simulink model "HVDC_MMC1_EMT"  (R2023b)
settings: Solver=ode23tb  StartTime=0.0  StopTime=10  MaxStep=Ts  RelTol=1e-3  EnableMultiTasking=on
PreLoadFcn:
  | HVDC_MMC_param
StartFcn:
  | tic
StopFcn:
  | toc
values from neighbouring files (symbols this model uses):
  acdcV = 1/(Vnom_dc/2*sqrt(3)/sqrt(2)/Vnom_sec)    [HVDC_MMC_param.m]
  C_PM = 1.758e-3    (= 0.001758)    [HVDC_MMC_param.m]
  Carm = 1.0*C_pm/n    (= 0.0002096)    [B2B_HVDC_MMC_Calc.m]    (also in HVDC_MMC_param.m = 4.88333333333e-05)
  DC_cable_C_shunt = 0.1e-6    (= 1e-07)    [HVDC_MMC_param.m]
  DC_cable_R_shunt = 1000    [HVDC_MMC_param.m]
  DCM = 1    [HVDC_MMC_param.m]
  Fn_filter = 1000    [B2B_HVDC_MMC_Calc.m]    (also in HVDC_MMC_param.m)
  Fnom = 50    [HVDC_MMC_param.m]
  HRM = 2    [HVDC_MMC_param.m]
  HrmOrd = N    (= 2)    [B2B_HVDC_MMC_Calc.m]    (also in HVDC_MMC_param.m)
  Ib_ac = (2/3)*Pnom/Vb_ac    [HVDC_MMC_param.m]
  Ib_dc = Pnom/Vb_dc    (= 1501.5015015)    [HVDC_MMC_param.m]
  Ki_CCSC = 50    [HVDC_MMC_param.m]
  Ki_Ireg = 6    [HVDC_MMC_param.m]
  Ki_Preg = 1.0    (= 1)    [HVDC_MMC_param.m]
  Ki_Qreg = 1.0    (= 1)    [HVDC_MMC_param.m]
  Ki_VDCreg = 100    [HVDC_MMC_param.m]
  Kp_CCSC = 0.8    [HVDC_MMC_param.m]
  Kp_Ireg = 0.6    [HVDC_MMC_param.m]
  Kp_Preg = 0.5/3    (= 0.166666666667)    [HVDC_MMC_param.m]
  Kp_Qreg = 0.5/3    (= 0.166666666667)    [HVDC_MMC_param.m]
  Kp_VDCreg = 4    [HVDC_MMC_param.m]
  L_cable = 15e-3    (= 0.015)    [HVDC_MMC_param.m]
  Larm = Larm_pu*(Zb_ac/w)    [HVDC_MMC_param.m]
  Lff = Larm_pu/2+Lxfo    (= 0.195)    [HVDC_MMC_param.m]
  Limits_Ireg = [ 2.0  -2.0]    [HVDC_MMC_param.m]
  Limits_Preg = [ 1.2, 0.8 ]    [HVDC_MMC_param.m]
  Limits_Qreg = [ 0.25, -0.25 ]    [HVDC_MMC_param.m]
  Limits_VDCreg = [ 2.0  -2.0]    [HVDC_MMC_param.m]
  Lxfo = 0.12    [HVDC_MMC_param.m]
  Pac = 0.9    [HVDC_MMC_param.m]
  Pnom = 1000e6    (= 1000000000)    [HVDC_MMC_param.m]
  Qac = 0.2    [HVDC_MMC_param.m]
  QCM = 0    [HVDC_MMC_param.m]
  R_cable = 0.5    [HVDC_MMC_param.m]
  Rarm = Rarm_pu*Zb_ac    [HVDC_MMC_param.m]
  Rff = Rarm_pu/2+Rxfo    (= 0.00375)    [HVDC_MMC_param.m]
  Rxfo = 0.003    [HVDC_MMC_param.m]
  Slope_Pref = 0.5    [HVDC_MMC_param.m]
  Slope_Qref = 0.5    [HVDC_MMC_param.m]
  Slope_Vdc_ref = Vnom_dc/5    (= 133200)    [HVDC_MMC_param.m]
  Tbrk1_On = 0.1    [HVDC_MMC_param.m]
  Tbrk2_On = 1.0    (= 1)    [HVDC_MMC_param.m]
  Tdeblock = 1.5    [HVDC_MMC_param.m]
  Tfault = 9999    [HVDC_MMC_param.m]
  Ton_Converter2 = 3    [HVDC_MMC_param.m]
  Ton_PQreg = 2    [HVDC_MMC_param.m]
  Ton_VDCreg = 1.5    [HVDC_MMC_param.m]
  Ts = Ts_Power    (= 5e-05)    [B2B_HVDC_MMC_Calc.m]    (also in HVDC_MMC_param.m)
  Ts_Control = Ts_Power    (= 5e-05)    [B2B_HVDC_MMC_Calc.m]    (also in HVDC_MMC_param.m)
  Ts_DQN = MultTs*Ts_Power    (= 5e-05)    [B2B_HVDC_MMC_Calc.m]    (also in HVDC_MMC_param.m)
  Ts_EMT = Ts    (= 5e-05)    [HVDC_MMC_param.m]
  Ts_Power = 1*50e-6    (= 5e-05)    [B2B_HVDC_MMC_Calc.m]    (also in HVDC_MMC_param.m)
  Vb_ac = sqrt(2/3)*Vnom_sec    [HVDC_MMC_param.m]
  Vb_dc = Vnom_dc    (= 666000)    [HVDC_MMC_param.m]
  Vc0_PM = 0    [HVDC_MMC_param.m]
  Vnom_dc = 2*Vnom_sec    (= 666000)    [HVDC_MMC_param.m]
  Vnom_prim = 333e3    (= 333000)    [HVDC_MMC_param.m]
  Vnom_sec = 333e3    (= 333000)    [HVDC_MMC_param.m]
  w = 2*pi*f    (= 314.159265359)    [B2B_HVDC_MMC_Calc.m]    (also in HVDC_MMC_param.m)
  Ws = 2*pi*Fnom    (= 314.159265359)    [HVDC_MMC_param.m]
  Zb_ac = Vb_ac/Ib_ac    [HVDC_MMC_param.m]
  Zeta_filter = 1    [B2B_HVDC_MMC_Calc.m]    (also in HVDC_MMC_param.m)
undefined symbols (not defined in the file or in its folder): DCss, DiscIntNeverNeededParam, gcbh, MT, sps_rtmsupport
libraries: DQN_Lib x37, simulink x35, spsCurrentMeasurementLib x24, powerlib_extras x21, slpidlib x14, spsSecondOrderFilterLib x14, spsVoltageMeasurementLib x10, spsSeriesRLCBranchLib x10, spsControlledVoltageSourceLib x9, spsHalfBridgeMMCmodel x7, spsGroundLib x4, spsParallelRLCBranchLib x4
(part 1 of 9)
settings Model: Creator=Pierre  LastModifiedBy=rober
settings SolverCC: ConcurrentTasks=on  AlgebraicLoopSolver=TrustRegion  AutoInsertRateTranBlk=on  InsertRTBMode=Never (minimum delay)
settings DataIOCC: SaveFormat=StructureWithTime  SignalLoggingSaveFormat=ModelDataLogs  SaveOutput=off  SignalLogging=off  DSMLogging=off  SaveTime=off  ReturnWorkspaceOutputs=off
settings OptimizationCC: DefaultParameterBehavior=Inlined  EnhancedBackFolding=on  PassReuseOutputArgsAs=Individual arguments  ExpressionDepthLimit=2147483647  OptimizeBlockOrder=speed  DifferentSizesBufferReuse=on  OptimizationCustomize=off  EfficientTunableParamExpr=on
settings DebuggingCC: UnderspecifiedInitializationDetection=Classic  MergeDetectMultiDrivingBlocksExec=none  SolverPrmCheckMsg=warning  ParameterTunabilityLossMsg=error  FcnCallInpInsideContextMsg=warning  UnconnectedInputMsg=warning  UnconnectedOutputMsg=warning  UnconnectedLineMsg=warning  AllowSymbolicDim=off  StateNameClashWarn=warning  SFUnexpectedBacktrackingDiag=warning  SFNoUnconditionalDefaultTransitionDiag=warning  SFExecutionAtInitializationDiag=none  ArithmeticOperatorsInVariantConditions=warning
settings ModelReferenceCC: EnableRefExpFcnMdlSchedulingChecks=on  PropagateSignalLabelsOutOfModel=off
settings SFSimCC: SimUseLocalCustomCode=off  MATLABDynamicMemAlloc=off  CustomCodeUndefinedFunction=UseInterfaceOnly
settings RTWCC: Description=Create Visual C/C++ Solution File for Embedded Coder  SystemTargetFile=ert.tlc  TemplateMakefile=RTW.MSVCBuild  GenerateReport=on  RTWUseLocalCustomCode=off  IncludeHyperlinkInReport=on  LaunchReport=on  GenerateTraceInfo=on  GenerateTraceReport=on  GenerateTraceReportSl=on  GenerateTraceReportSf=on  GenerateTraceReportEml=on  DLArmComputeVersion=19.05
settings CodeAppCC: ForceParamTrailComments=on  IgnoreCustomStorageClasses=off  OperatorAnnotations=on  SimulinkDataObjDesc=on  SFDataObjDesc=on  InsertBlockDesc=on
settings ERTTargetCC: GenerateSampleERTMain=on  InlinedParameterPlacement=NonHierarchical  ERTCustomFileTemplate=example_file_process.tlc
settings ConfigComp: CovMetricSettings=dw  CovSaveCumulativeToWorkspaceVar=on  CovSaveSingleToWorkspaceVar=on  CovExternalEMLEnable=off
settings SimscapeCC: SimscapeNormalizeSystem=off

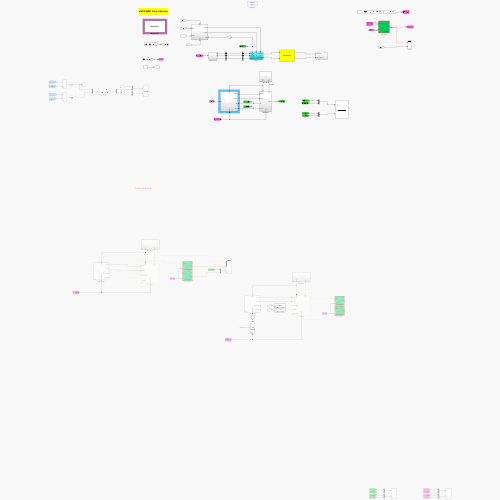
[thumbnail: Simulink's stored preview of the top-level diagram]
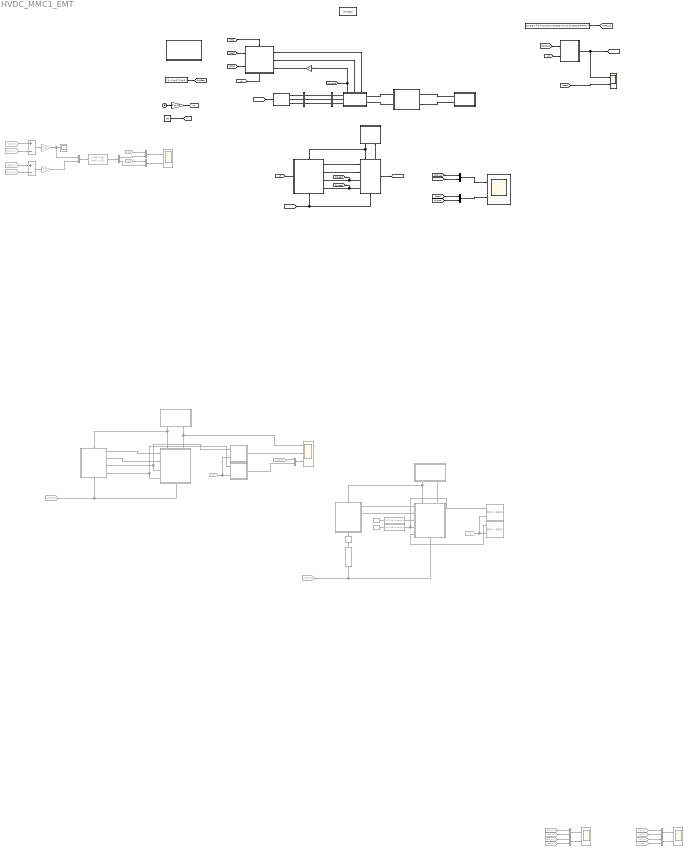
== system HVDC_MMC1_EMT ==
  note: HVDC-MMC Control System
  Add : Sum  Commented=on  Inputs=+-
  Add1 : Sum  Commented=on  Inputs=+-
  CTRL_DQN1 : Subsystem  Commented=on  mask{HarmOrd=HRM}
      mask prompts: HarmOrd "Harmonic order:"
      settings: PortSchema="{\"entries\":[{\"content\":{\"sides\":[{\"content\":{\"connectorIds\":[]},\"type\":\"ConnectorPlacement.EquallySpacedRectSide\",\"uuid\":\"0d082dcb-1cb9-4a87-98e5-35cd432a3a21\"},{\"content\":{\"connectorIds\":[\"Out1\",\"Out2\",\"In3\",\"In4\"],\"side\":\"RIGHT\"},\"type\":\"ConnectorPlacement.EquallySpacedRectSide\",\"uuid\":\"d6c14327-33b3-4ee6-a1e0-7651c9b95832\"},{\"content\":{\"connectorIds\":[\"In1\"],\"side\":\"TOP\"},\"type\":\"ConnectorPlacement.EquallySpacedRectSide\",\"uuid\":\"6be6102f-c019-430a-8225-c31cf73f3a4d\"},{\"content\":{\"connectorIds\":[\"In2\"],\"side\":\"BOTTOM\"},\"type\":\"ConnectorPlacement.EquallySpacedRectSide\",\"uuid\":\"0001f10d-d46a-487c-af5a-06cf58c2ee1d\"}]},\"type\":\"ConnectorPlacement.EquallySpacedConnector\",\"uuid\":\"6102694e-9904-4f4a-845e-781e1c53da4b\"}],\"packageUris\":[\"http://schema.mathworks.com/mf0/Connector/R2020b\"],\"version\":\"1.0\"}"
  CTRL_DQN3 : Subsystem  Commented=on  mask{HarmOrd=HRM}
      mask prompts: HarmOrd "Harmonic order:"
      settings: PortSchema="{\"entries\":[{\"content\":{\"sides\":[{\"content\":{\"connectorIds\":[]},\"type\":\"ConnectorPlacement.EquallySpacedRectSide\",\"uuid\":\"0d082dcb-1cb9-4a87-98e5-35cd432a3a21\"},{\"content\":{\"connectorIds\":[\"Out1\",\"Out2\",\"In3\",\"In4\"],\"side\":\"RIGHT\"},\"type\":\"ConnectorPlacement.EquallySpacedRectSide\",\"uuid\":\"d6c14327-33b3-4ee6-a1e0-7651c9b95832\"},{\"content\":{\"connectorIds\":[\"In1\"],\"side\":\"TOP\"},\"type\":\"ConnectorPlacement.EquallySpacedRectSide\",\"uuid\":\"6be6102f-c019-430a-8225-c31cf73f3a4d\"},{\"content\":{\"connectorIds\":[\"In2\"],\"side\":\"BOTTOM\"},\"type\":\"ConnectorPlacement.EquallySpacedRectSide\",\"uuid\":\"0001f10d-d46a-487c-af5a-06cf58c2ee1d\"}]},\"type\":\"ConnectorPlacement.EquallySpacedConnector\",\"uuid\":\"6102694e-9904-4f4a-845e-781e1c53da4b\"}],\"packageUris\":[\"http://schema.mathworks.com/mf0/Connector/R2020b\"],\"version\":\"1.0\"}"
  Clock : Clock
  Constant1 : Constant  Value="[ 0  -2*pi/3  2*pi/3 ]"  SampleTime=-1
  Constant3 : Constant  Value=complex( [[ 0 Vnom_prim*sqrt(2/3); 0 0; 0 0] zeros(3,HRM-1) ])
  DC Circuit1 : Subsystem
      mask Display: disp('DC circuit')
  DC circuit : StateSpace  Commented=on  A=DCss.A  B=DCss.B  C=DCss.C  D=DCss.D  InitialCondition=DCss.x0
  DC_ABC : Subsystem
      settings: PortSchema="{\"entries\":[{\"content\":{\"sides\":[{\"content\":{\"connectorIds\":[]},\"type\":\"ConnectorPlacement.EquallySpacedRectSide\",\"uuid\":\"5f9f81b4-6131-4450-96fc-72212a851b46\"},{\"content\":{\"connectorIds\":[],\"side\":\"RIGHT\"},\"type\":\"ConnectorPlacement.EquallySpacedRectSide\",\"uuid\":\"0f788077-5580-4ce6-8a1f-7a09e9370e5a\"},{\"content\":{\"connectorIds\":[],\"side\":\"TOP\"},\"type\":\"ConnectorPlacement.EquallySpacedRectSide\",\"uuid\":\"37f0a42c-2dd3-49bf-9631-153ec1fd1df0\"},{\"content\":{\"connectorIds\":[\"In1\",\"Out1\"],\"side\":\"BOTTOM\"},\"type\":\"ConnectorPlacement.EquallySpacedRectSide\",\"uuid\":\"4a78dd89-41c9-4db8-9bc2-9f49ec3f0c10\"}]},\"type\":\"ConnectorPlacement.EquallySpacedConnector\",\"uuid\":\"5112b42b-f0ed-441a-b745-2a1f4f5dce4a\"}],\"packageUris\":[\"http://schema.mathworks.com/mf0/Connector/19700101\"],\"version\":\"1.0\"}"
  DC_ABC1 : Subsystem  Commented=on
      settings: PortSchema="{\"entries\":[{\"content\":{\"sides\":[{\"content\":{\"connectorIds\":[]},\"type\":\"ConnectorPlacement.EquallySpacedRectSide\",\"uuid\":\"5f9f81b4-6131-4450-96fc-72212a851b46\"},{\"content\":{\"connectorIds\":[],\"side\":\"RIGHT\"},\"type\":\"ConnectorPlacement.EquallySpacedRectSide\",\"uuid\":\"0f788077-5580-4ce6-8a1f-7a09e9370e5a\"},{\"content\":{\"connectorIds\":[],\"side\":\"TOP\"},\"type\":\"ConnectorPlacement.EquallySpacedRectSide\",\"uuid\":\"37f0a42c-2dd3-49bf-9631-153ec1fd1df0\"},{\"content\":{\"connectorIds\":[\"In1\",\"Out1\"],\"side\":\"BOTTOM\"},\"type\":\"ConnectorPlacement.EquallySpacedRectSide\",\"uuid\":\"4a78dd89-41c9-4db8-9bc2-9f49ec3f0c10\"}]},\"type\":\"ConnectorPlacement.EquallySpacedConnector\",\"uuid\":\"5112b42b-f0ed-441a-b745-2a1f4f5dce4a\"}],\"packageUris\":[\"http://schema.mathworks.com/mf0/Connector/R2020b\"],\"version\":\"1.0\"}"
  DC_ABC2 : Subsystem  Commented=on
      settings: PortSchema="{\"entries\":[{\"content\":{\"sides\":[{\"content\":{\"connectorIds\":[]},\"type\":\"ConnectorPlacement.EquallySpacedRectSide\",\"uuid\":\"5f9f81b4-6131-4450-96fc-72212a851b46\"},{\"content\":{\"connectorIds\":[],\"side\":\"RIGHT\"},\"type\":\"ConnectorPlacement.EquallySpacedRectSide\",\"uuid\":\"0f788077-5580-4ce6-8a1f-7a09e9370e5a\"},{\"content\":{\"connectorIds\":[],\"side\":\"TOP\"},\"type\":\"ConnectorPlacement.EquallySpacedRectSide\",\"uuid\":\"37f0a42c-2dd3-49bf-9631-153ec1fd1df0\"},{\"content\":{\"connectorIds\":[\"In1\",\"Out1\"],\"side\":\"BOTTOM\"},\"type\":\"ConnectorPlacement.EquallySpacedRectSide\",\"uuid\":\"4a78dd89-41c9-4db8-9bc2-9f49ec3f0c10\"}]},\"type\":\"ConnectorPlacement.EquallySpacedConnector\",\"uuid\":\"5112b42b-f0ed-441a-b745-2a1f4f5dce4a\"}],\"packageUris\":[\"http://schema.mathworks.com/mf0/Connector/R2020b\"],\"version\":\"1.0\"}"
  DQn->ABC : MATLAB Function  TreatAsAtomicUnit=on  SystemSampleTime=Ts  mask{N=HRM}
      mask prompts: N "Harmonic order:"
  DQn->ABC1 : DQN_Lib/DQn->ABC6  Commented=on  N=HrmOrd
  DQn->ABC2 : MATLAB Function  Commented=on  TreatAsAtomicUnit=on  SystemSampleTime=Ts  mask{N=HrmOrd}
      mask prompts: N "Harmonic order:"
  DQn->ABC3 : MATLAB Function  Commented=on  TreatAsAtomicUnit=on  SystemSampleTime=Ts  mask{N=HrmOrd}
      mask prompts: N "Harmonic order:"
  DQn->ABC9 : DQN_Lib/DQn->ABC6  Commented=on  N=HrmOrd
  Demux : Demux  Commented=on  Outputs=2
  From : From  Commented=on  GotoTag=Vdc1  TagVisibility=global
  From1 : From  Commented=on  GotoTag=wt  TagVisibility=global
  From17 : From  Commented=on  GotoTag=Idc_plus  TagVisibility=global
  From19 : From  Commented=on  GotoTag=Idc_minus  TagVisibility=global
  From20 : From  Commented=on  GotoTag=Irec_minus  TagVisibility=global
  From23 : From  Commented=on  GotoTag=Irec_plus  TagVisibility=global
  From24 : From  Commented=on  GotoTag=Vdc2  TagVisibility=global
  From27 : From  Commented=on  GotoTag=Idiff_d2_c  TagVisibility=global
  From30 : From  Commented=on  GotoTag=wt  TagVisibility=global
  From52 : From  Commented=on  GotoTag=Idiff_q2_c  TagVisibility=global
  From53 : From  Commented=on  GotoTag=Idiff_q2  TagVisibility=global
  From55 : From  Commented=on  GotoTag=Idiff_d2  TagVisibility=global
  From56 : From  Commented=on  GotoTag=Md2_c  TagVisibility=global
  From57 : From  Commented=on  GotoTag=Mq2_c  TagVisibility=global
  From58 : From  Commented=on  GotoTag=Md2  TagVisibility=global
  From59 : From  Commented=on  GotoTag=Mq2  TagVisibility=global
  From6 : From  Commented=on  GotoTag=VSRC_C
  From7 : From  Commented=on  GotoTag=Id_abc
  From9 : From  Commented=on  GotoTag=VSRC_C
  Gain : Gain  Gain=2*pi*50
  Gain1 : Gain  Gain=-1
  Gain2 : Gain  Commented=on  Gain=-0.5
  Gain3 : Gain  Commented=on  Gain=0.5
  MATLAB Function1 : DQN_Lib/MATLAB Function4  Commented=on  SystemSampleTime=-1  VariantActivationTime=update diagram  AllowFlexibleInterface=on  Latency=0  AutoFrameSizeCalculation=off
  MATLAB Function2 : DQN_Lib/MATLAB Function4  Commented=on  SystemSampleTime=-1  VariantActivationTime=update diagram  AllowFlexibleInterface=on  Latency=0  AutoFrameSizeCalculation=off
  MATLAB Function9 : DQN_Lib/MATLAB Function4  Commented=on  SystemSampleTime=-1  VariantActivationTime=update diagram  AllowFlexibleInterface=on  Latency=0  AutoFrameSizeCalculation=off
  MMC : Subsystem
      settings: PortSchema="{\"entries\":[{\"content\":{\"sides\":[{\"content\":{\"connectorIds\":[\"LConn1\",\"LConn2\",\"LConn3\"]},\"type\":\"ConnectorPlacement.EquallySpacedRectSide\",\"uuid\":\"74479f40-f186-427a-9533-cd542da214a9\"},{\"content\":{\"connectorIds\":[\"RConn1\",\"RConn2\"],\"side\":\"RIGHT\"},\"type\":\"ConnectorPlacement.EquallySpacedRectSide\",\"uuid\":\"af2aab5a-8cfc-47b9-a3d5-dec541285526\"},{\"content\":{\"connectorIds\":[\"Out1\",\"In1\",\"In2\"],\"side\":\"TOP\"},\"type\":\"ConnectorPlacement.EquallySpacedRectSide\",\"uuid\":\"775fe849-b2f4-496e-a9c1-c2c8ec805134\"}]},\"type\":\"ConnectorPlacement.EquallySpacedConnector\",\"uuid\":\"59d7b4d4-c63b-4498-b4b5-ac9188fab092\"}],\"packageUris\":[\"http://schema.mathworks.com/mf0/Connector/R2020b\"],\"version\":\"1.0\"}"
  MMC_ABC : Subsystem
      settings: PortSchema="{\"entries\":[{\"content\":{\"sides\":[{\"content\":{\"connectorIds\":[\"In1\",\"In2\",\"Out3\",\"Out4\"]},\"type\":\"ConnectorPlacement.EquallySpacedRectSide\",\"uuid\":\"684906a0-21fb-41a6-b3c5-f77045d253ac\"},{\"content\":{\"connectorIds\":[\"Out1\"],\"side\":\"RIGHT\"},\"type\":\"ConnectorPlacement.EquallySpacedRectSide\",\"uuid\":\"9d85a733-ae48-4655-9ff6-63838a16e886\"},{\"content\":{\"connectorIds\":[\"In3\",\"Out2\"],\"side\":\"TOP\"},\"type\":\"ConnectorPlacement.EquallySpacedRectSide\",\"uuid\":\"d076c62e-607a-4519-bbe3-5591fb02f9d6\"},{\"content\":{\"connectorIds\":[\"In4\"],\"side\":\"BOTTOM\"},\"type\":\"ConnectorPlacement.EquallySpacedRectSide\",\"uuid\":\"e22e3e72-7b47-4480-8e5d-6e636dd9340b\"}]},\"type\":\"ConnectorPlacement.EquallySpacedConnector\",\"uuid\":\"6c134aa3-44e6-4e9e-9485-00d5bee37874\"}],\"packageUris\":[\"http://schema.mathworks.com/mf0/Connector/R2020b\"],\"version\":\"1.0\"}"
  MMC_DQN : Subsystem  Commented=on  mask{HrmOrd=HRM, AngFreq=Ws, TimeStep=Ts_DQN}
      mask prompts: HrmOrd "Harmonic order:"; AngFreq "Angular frequency (rad/s):"; TimeStep "Time step (s):"
      settings: PortSchema="{\"entries\":[{\"content\":{\"sides\":[{\"content\":{\"connectorIds\":[\"In1\",\"In2\",\"Out2\",\"Out3\",\"Out4\"]},\"type\":\"ConnectorPlacement.EquallySpacedRectSide\",\"uuid\":\"f639eebb-f91d-4893-aa5c-614953e50141\"},{\"content\":{\"connectorIds\":[],\"side\":\"RIGHT\"},\"type\":\"ConnectorPlacement.EquallySpacedRectSide\",\"uuid\":\"a5873f74-8648-46cb-b48a-fb2ca776885a\"},{\"content\":{\"connectorIds\":[\"In3\",\"Out1\"],\"side\":\"TOP\"},\"type\":\"ConnectorPlacement.EquallySpacedRectSide\",\"uuid\":\"7f3a2d41-300e-41de-a385-bf2dc4de27d8\"},{\"content\":{\"connectorIds\":[\"In4\"],\"side\":\"BOTTOM\"},\"type\":\"ConnectorPlacement.EquallySpacedRectSide\",\"uuid\":\"dc3c6aa9-7c8d-4c08-aa50-6213fc2a18de\"}]},\"type\":\"ConnectorPlacement.EquallySpacedConnector\",\"uuid\":\"a22dadcf-e226-432e-bcde-0bea34be45da\"}],\"packageUris\":[\"http://schema.mathworks.com/mf0/Connector/R2020b\"],\"version\":\"1.0\"}"
  MMC_DQN1 : Subsystem  Commented=on  mask{HrmOrd=HRM, AngFreq=Ws, TimeStep=Ts_DQN}
      mask prompts: HrmOrd "Harmonic order:"; AngFreq "Angular frequency (rad/s):"; TimeStep "Time step (s):"
      settings: PortSchema="{\"entries\":[{\"content\":{\"sides\":[{\"content\":{\"connectorIds\":[\"In1\",\"In2\",\"Out2\",\"Out3\"]},\"type\":\"ConnectorPlacement.EquallySpacedRectSide\",\"uuid\":\"f639eebb-f91d-4893-aa5c-614953e50141\"},{\"content\":{\"side\":\"RIGHT\"},\"type\":\"ConnectorPlacement.EquallySpacedRectSide\",\"uuid\":\"a5873f74-8648-46cb-b48a-fb2ca776885a\"},{\"content\":{\"connectorIds\":[\"In3\",\"Out1\"],\"side\":\"TOP\"},\"type\":\"ConnectorPlacement.EquallySpacedRectSide\",\"uuid\":\"7f3a2d41-300e-41de-a385-bf2dc4de27d8\"},{\"content\":{\"connectorIds\":[\"In4\"],\"side\":\"BOTTOM\"},\"type\":\"ConnectorPlacement.EquallySpacedRectSide\",\"uuid\":\"dc3c6aa9-7c8d-4c08-aa50-6213fc2a18de\"}]},\"type\":\"ConnectorPlacement.EquallySpacedConnector\",\"uuid\":\"a22dadcf-e226-432e-bcde-0bea34be45da\"}],\"packageUris\":[\"http://schema.mathworks.com/mf0/Connector/R2020b\"],\"version\":\"1.0\"}"
  Mux{,1..3,15..18} (8 alike) : Mux  Commented=on  Inputs=2
  Mux4 : Mux  Inputs=2
  Mux5 : Mux  Inputs=2
  Pi1 : Constant  Value=50  OutDataTypeStr=Inherit: Inherit via back propagation
  Reshape : Reshape  Commented=on
  Reshape1 : Reshape  Commented=on
  Reshape2 : Reshape  Commented=on
  Scope : Scope  NumInputPorts=2
  Scope1 : Scope  NumInputPorts=2
  Scope10 : Scope  Commented=on  NumInputPorts=2
  Scope2 : Scope  Commented=on  NumInputPorts=3
  Scope3 : Scope  Commented=on
  Scope4 : Scope  Commented=on  NumInputPorts=2
  Scope9 : Scope  Commented=on  NumInputPorts=2
  Sequencer : Subsystem
      mask Display: disp('Sequencer')
  Subsystem : Subsystem
      settings: PortSchema="{\"entries\":[{\"content\":{\"sides\":[{\"content\":{\"connectorIds\":[\"In1\"]},\"type\":\"ConnectorPlacement.EquallySpacedRectSide\",\"uuid\":\"0eb80377-11e9-4327-8c94-fb94b1ae678e\"},{\"content\":{\"connectorIds\":[\"Out1\",\"Out2\",\"In4\",\"In5\"],\"side\":\"RIGHT\"},\"type\":\"ConnectorPlacement.EquallySpacedRectSide\",\"uuid\":\"6596dc6b-6b23-47fc-bea2-6996abd2ba15\"},{\"content\":{\"connectorIds\":[\"In2\"],\"side\":\"TOP\"},\"type\":\"ConnectorPlacement.EquallySpacedRectSide\",\"uuid\":\"8e21476a-42ed-42f6-8dc5-d6cd1acd5e6a\"},{\"content\":{\"connectorIds\":[\"In3\"],\"side\":\"BOTTOM\"},\"type\":\"ConnectorPlacement.EquallySpacedRectSide\",\"uuid\":\"64f4f9aa-7403-4df9-a838-1dcd5c8e1624\"}]},\"type\":\"ConnectorPlacement.EquallySpacedConnector\",\"uuid\":\"bea88ec7-c79f-4685-875b-b84ad23b5423\"}],\"packageUris\":[\"http://schema.mathworks.com/mf0/Connector/R2020b\"],\"version\":\"1.0\"}"
  Subsystem1 : Subsystem
  Subsystem2 : Subsystem
      settings: PortSchema="{\"entries\":[{\"content\":{\"sides\":[{\"content\":{\"connectorIds\":[\"In1\",\"In2\"]},\"type\":\"ConnectorPlacement.EquallySpacedRectSide\",\"uuid\":\"0eb80377-11e9-4327-8c94-fb94b1ae678e\"},{\"content\":{\"connectorIds\":[\"Out1\",\"Out2\",\"In5\"],\"side\":\"RIGHT\"},\"type\":\"ConnectorPlacement.EquallySpacedRectSide\",\"uuid\":\"6596dc6b-6b23-47fc-bea2-6996abd2ba15\"},{\"content\":{\"connectorIds\":[\"In3\"],\"side\":\"TOP\"},\"type\":\"ConnectorPlacement.EquallySpacedRectSide\",\"uuid\":\"8e21476a-42ed-42f6-8dc5-d6cd1acd5e6a\"},{\"content\":{\"connectorIds\":[\"In4\"],\"side\":\"BOTTOM\"},\"type\":\"ConnectorPlacement.EquallySpacedRectSide\",\"uuid\":\"64f4f9aa-7403-4df9-a838-1dcd5c8e1624\"}]},\"type\":\"ConnectorPlacement.EquallySpacedConnector\",\"uuid\":\"bea88ec7-c79f-4685-875b-b84ad23b5423\"}],\"packageUris\":[\"http://schema.mathworks.com/mf0/Connector/R2020b\"],\"version\":\"1.0\"}"
  Voltage source : Subsystem
  conv : spsThreePhaseVIMeasurementLib/Three-Phase V-I Measurement  VoltageMeasurement=phase-to-ground  SetLabelV=on  LabelV=Vconv  Vpu=off  VpuLL=off  CurrentMeasurement=no  SetLabelI=on  LabelI=Isec  Ipu=off  Pbase=100e6  Vbase=500e3  OutputType=Complex  PhasorSimulation=off  PSBequivalent=0
  powergui : spspowerguiLib/powergui  Priority=1  SimulationMode=Discrete  SampleTime=Ts  frequency=60  Iterations=50  frequencyindice=0  Pbase=100e6  ErrMax=1e-4  UnitsV=kV  UnitsW=MW  buscounter=0  FunctionMessages=off  echomessages=off  EnableUseOfTLC=off  CurrentSourceSwitches=off  DisableSnubberDevices=off  DisableRonSwitches=off  DisableVfSwitches=off  DisplayEquations=off  AutomaticDiscreteSolvers=off  SolverType=Tustin/Backward Euler (TBE)  Interpol=off  ExternalGateDelay=off  methode=off  Ts=100  x0status=blocks  SPID=off  SwTol=0  HookPort=off  NonlinearTolerance=1e-4  nMaxIteration=100  ContinueOnMaxIteration=off  RestoreLinks=warning  ResistiveCurrentMeasurement=off  Frange=[0:2:500]  Ylog=off  Xlog=on  ShowGrid=off  save=off  variable=ZData  structure=ScopeData1  ZoomFFT=off  StartTime=9  cycles=100  DisplayStyle=1  fundamental=50  FreqAxis=off  MaxFrequency=100  frequencyindicesteady=1  RmsSteady=1  display=off
  sec : spsThreePhaseVIMeasurementLib/Three-Phase V-I Measurement  VoltageMeasurement=phase-to-ground  SetLabelV=on  LabelV=Vsec  Vpu=off  VpuLL=off  CurrentMeasurement=yes  SetLabelI=on  LabelI=Isec  Ipu=off  Pbase=100e6  Vbase=500e3  OutputType=Complex  PhasorSimulation=off  PSBequivalent=0
  tag scope: PosSeq=global, f=global, wt=global
  wires:
  Pi1/1 -> [f]
  Gain/1 -> [wt]
  Clock/1 -> Gain/1
  Constant1/1 -> [PosSeq]
  Mux15/1 -> Scope9/1
  Mux16/1 -> Scope9/2
  From55/1 -> Mux15/2
  From27/1 -> Mux15/1
  From53/1 -> Mux16/2
  From52/1 -> Mux16/1
  Mux18/1 -> Scope10/2
  From56/1 -> Mux17/1
  From59/1 -> Mux18/2
  From58/1 -> Mux17/2
  Mux17/1 -> Scope10/1
  From57/1 -> Mux18/1
  [Vsec] -> Scope/2
  [wt] -> DQn->ABC/2(tho)  "theta"
  Constant3/1 -> [VSRC_C]
  [VSRC_C] -> DQn->ABC/1(Xdcpnz_c)  "[N+1,18 (6+6+6)]"
  DQn->ABC/1(Xabc) -> Scope/1, [Vsec_ABC]  "Mac_EMT"
  MMC_ABC/4(Iconv1) -> [Ic_abc], Subsystem/5(Iconv)
  Subsystem/1("{m_dq1}") -> MMC_ABC/1(m_dq1)
  [Vsec_ABC] -> Subsystem/3(Vsec), MMC_ABC/4(Vsec)
  DC_ABC/1(Vdc1) -> Subsystem/2(Vdc), MMC_ABC/3(Vdc)
  [wt] -> Subsystem/1(wt)
  Subsystem/2("{m_dq2}") -> MMC_ABC/2(m_dq2)
  MMC_ABC/2(Idc) -> DC_ABC/1(Idc1)  "Idc_ABC"
  MMC_ABC/3(Id) -> [Id_abc], Subsystem/4(Idiff)
  CTRL_DQN3/1(m_dq1) -> MMC_DQN/1(m_dq1)
  ? -> ?
  DC_ABC1/1(Vdc1) -> CTRL_DQN3/1(Vdc), MMC_DQN/3(Vdc)
  CTRL_DQN3/2(m_dq2) -> MMC_DQN/2(m_dq2)
  From30/1 -> DQn->ABC1/2, DQn->ABC9/2
  From6/1 -> MATLAB Function2/1, MMC_DQN/4(Vs_DQN)
  MMC_DQN/4(Vconv_DQN) -> DQn->ABC1/1
  MMC_DQN/3(Id_DQN) -> DQn->ABC9/1, MATLAB Function1/1
  MMC_DQN/2(Iconv_DQN) -> MATLAB Function9/1
  MMC_DQN/1(Idc) -> DC_ABC1/1(Idc1)
  Subsystem2/2("{m_dq2}") -> MMC/1(m_dq2)
  [Isec] -> Subsystem2/2(Iconv)
  Subsystem2/1("{m_dq1}") -> MMC/2(m_dq1)
  MMC/1(Id_abc) -> Gain1/1, [Id_emt]
  [Vdc1] -> Subsystem2/3(Vdc)
  [Vsec] -> Subsystem2/1(Vsec)
  Gain1/1 -> Subsystem2/5(Idiff)
  [wt] -> Subsystem2/4(wt)
  [Vsec_ABC] -> Voltage source/1(In1)
  MATLAB Function9/1 -> Reshape/1
  MATLAB Function1/1 -> Reshape1/1
  MATLAB Function2/1 -> Reshape2/1
  Reshape2/1 -> CTRL_DQN3/2(Vs_DQN)
  CTRL_DQN1/1(m_dq1) -> MMC_DQN1/1(m_dq1)
  DC_ABC2/1(Vdc1) -> CTRL_DQN1/1(Vdc), MMC_DQN1/3(Vdc)
  CTRL_DQN1/2(m_dq2) -> MMC_DQN1/2(m_dq2)
  MMC_DQN1/1(Idc) -> DC_ABC2/1(Idc1), Scope2/1
  From9/1 -> MMC_DQN1/4(Vs_DQN), CTRL_DQN1/2(Vs_DQN)
  From1/1 -> DQn->ABC2/2(tho), DQn->ABC3/2(tho)
  MMC_DQN1/2(Iconv_DQN) -> DQn->ABC3/1(Xdcpnz_c), CTRL_DQN1/3(Iconv_DQN)
  MMC_DQN1/3(Id_DQN) -> DQn->ABC2/1(Xdcpnz_c), CTRL_DQN1/4(Id_DQN)
  DQn->ABC2/1(Xabc) -> Mux/2
  DQn->ABC3/1(Xabc) -> Scope2/2
  Mux/1 -> Scope2/3
  From7/1 -> Mux/1
  Mux1/1 -> DC circuit/1
  DC circuit/1 -> Demux/1
  From19/1 -> Add/2
  Add/1 -> Gain2/1
  Gain2/1 -> Mux1/1, Scope3/1
  From17/1 -> Add/1
  From23/1 -> Add1/1
  From20/1 -> Add1/2
  Add1/1 -> Gain3/1
  Gain3/1 -> Mux1/2
  Mux2/1 -> Scope4/1
  Mux3/1 -> Scope4/2
  From/1 -> Mux2/1
  Demux/1 -> Mux2/2
  From24/1 -> Mux3/1
  Demux/2 -> Mux3/2
  MMC_ABC/1(Vconv) -> [Vconv_abc]
  [Vconv_abc] -> Mux4/2
  [Ic_abc] -> Mux5/2
  [Isec] -> Mux5/1
  [Vconv] -> Mux4/1
  Mux4/1 -> Scope1/1
  Mux5/1 -> Scope1/2
  connections:
  sec/LConn1 -- conv/RConn1
  Voltage source/RConn3 -- sec/RConn3
  MMC/LConn3 -- conv/LConn3
  sec/LConn3 -- conv/RConn3
  sec/LConn2 -- conv/RConn2
  MMC/LConn1 -- conv/LConn1
  Voltage source/RConn1 -- sec/RConn1
  Voltage source/RConn2 -- sec/RConn2
  MMC/LConn2 -- conv/LConn2
  DC Circuit1/LConn1 -- MMC/RConn1
  DC Circuit1/LConn2 -- MMC/RConn2
  DC Circuit1/RConn1 -- Subsystem1/LConn1
  DC Circuit1/RConn2 -- Subsystem1/LConn2

== system HVDC_MMC1_EMT/CTRL_DQN1 ==
  Vdc : Inport
  Vs_DQN : Inport  Port=2
  Iconv_DQN : Inport  Port=3
  Id_DQN : Inport  Port=4
  I->pu1 : Gain  Gain=1/Ib_ac  SaturateOnIntegerOverflow=on  OutDataTypeStr=Inherit: Same as input  ParamDataTypeStr=Inherit: Same as input
  I->pu13 : Gain  Gain=1/Vb_ac  SaturateOnIntegerOverflow=on  OutDataTypeStr=Inherit: Same as input  ParamDataTypeStr=Inherit: Same as input
  I->pu2 : Gain  Gain=1/Ib_ac  SaturateOnIntegerOverflow=on  OutDataTypeStr=Inherit: Same as input  ParamDataTypeStr=Inherit: Same as input
  MATLAB Function1 : DQN_Lib/MATLAB Function4  SystemSampleTime=-1  VariantActivationTime=update diagram  AllowFlexibleInterface=on  Latency=0  AutoFrameSizeCalculation=off
  MATLAB Function4 : DQN_Lib/MATLAB Function4  SystemSampleTime=-1  VariantActivationTime=update diagram  AllowFlexibleInterface=on  Latency=0  AutoFrameSizeCalculation=off
  MATLAB Function9 : DQN_Lib/MATLAB Function4  SystemSampleTime=-1  VariantActivationTime=update diagram  AllowFlexibleInterface=on  Latency=0  AutoFrameSizeCalculation=off
  Mux1 : Mux  Inputs=2
  Mux3 : Mux  Inputs=2
  Mux4 : Mux  Inputs=2
  Reshape : Reshape
  Reshape1 : Reshape
  Reshape4 : Reshape
  Selector1 : Selector  InputPortWidth=HrmOrd+1  IndexOptions=Index vector (dialog)  Indices=3  OutputSizes=1
  Selector{6..7,9..10} (4 alike) : Selector  InputPortWidth=HrmOrd+1  IndexOptions=Index vector (dialog)  Indices=2  OutputSizes=1
  Selector2 : Selector  InputPortWidth=HrmOrd+1  IndexOptions=Index vector (dialog)  Indices=3  OutputSizes=1
  Subsystem : DQN_Lib/Subsystem  N=HrmOrd
  Subsystem1 : Subsystem  Commented=on
  Subsystem2 : Subsystem  mask{Ts=Ts_DQN, Fnom=Fnom, acdcV=acdcV, Fn_filter=Fn_filter, Zeta_filter=Zeta_filter, Kp_Preg=Kp_Preg, Ki_Preg=Ki_Preg, Limits_Preg_1=Limits_Preg(1), Limits_Preg_2=Limits_Preg(2), Kp_Qreg=Kp_Qreg, Ki_Qreg=Ki_Qreg, Limits_Qreg_1=Limits_Qreg(1), Limits_Qreg_2=Limits_Qreg(2), Kp_VDCreg=Kp_VDCreg, Ki_VDCreg=Ki_VDCreg, Limits_VDCreg_1=Limits_VDCreg(1), Limits_VDCreg_2=Limits_VDCreg(2), Kp_Ireg=Kp_Ireg, Ki_Ireg=Ki_Ireg, Limits_Ireg=Limits_Ireg, Rff=Rff, Lff=Lff, Kp_CCSC=Kp_CCSC, Ki_CCSC=Ki_CCSC}
      mask prompts: Ts "Sample time:"; Fnom "Fundamental frequency (Hz):"; Fn_filter "Natural frequency fn (Hz):"; Zeta_filter "Damping ratio Zeta"; Kp_Preg "Proportional (P):"; Ki_Preg "Integral (I):"; Limits_Preg_1 "Upper limit:"; Limits_Preg_2 "Lower limit:"; Kp_Qreg "Proportional (P):"; Ki_Qreg "Integral (I):"; Limits_Qreg_1 "Upper limit:"; Limits_Qreg_2 "Lower limit:"; Kp_VDCreg "Proportional (P):"; Ki_VDCreg "Integral (I):"; Limits_VDCreg_1 "Upper limit:"; Limits_VDCreg_2 "Lower limit:"; Kp_Ireg "Proportional (P):"; Ki_Ireg "Integral (I):"; Limits_Ireg "Output limits:"; Kp_CCSC "Proportional (P):"; Ki_CCSC "Integral (I):"
      mask DialogControl Container6 Prompt: General
      mask DialogControl Container14 Prompt: Filter
      mask DialogControl Container14_copy Prompt: Active power regulator
      mask DialogControl Container14_copy_copy Prompt: Reactive power regulator
      mask DialogControl Container14_copy_copy_copy Prompt: DC voltage regulator
      mask DialogControl Container14_copy_copy_copy_copy Prompt: Current regulator
      mask DialogControl Container14_copy_copy_copy_copy_copy Prompt: CCSC
  Subsystem4 : DQN_Lib/Subsystem  N=HrmOrd
  Subsystem5 : DQN_Lib/Subsystem  N=HrmOrd
  V->pu1 : Gain  Gain=1/Vb_ac  SaturateOnIntegerOverflow=on  OutDataTypeStr=Inherit: Same as input  ParamDataTypeStr=Inherit: Same as input
  m_dq1 : Outport
  m_dq2 : Outport  Port=2
  wires:
  Subsystem5/4 -> Selector10/1
  Subsystem4/1 -> Selector6/1
  Subsystem4/4 -> Selector7/1
  Subsystem5/1 -> Selector9/1
  V->pu1/1 -> Subsystem5/1
  Reshape4/1 -> V->pu1/1
  Vdc/1 -> I->pu13/1
  Subsystem2/1(m_dq1) -> m_dq1/1
  I->pu2/1 -> Subsystem4/1
  I->pu13/1 -> Subsystem2/1(Vdc)
  Mux4/1 -> Subsystem2/2(Vs_dq1)
  Mux3/1 -> Subsystem2/3(Iconv_dq1)
  Subsystem/5 -> Selector2/1
  I->pu1/1 -> Subsystem/1
  Selector1/1 -> Mux1/1
  Selector2/1 -> Mux1/2
  Mux1/1 -> Subsystem2/4(Id_dq2)
  Subsystem/2 -> Selector1/1
  [PSCC_On] -> Subsystem2/8(PQreg_On1)
  [PQreg_On] -> Subsystem2/5(PQreg_On)
  [VDCreg_On] -> Subsystem2/6(VDCreg_On)
  Selector9/1 -> Mux4/1
  Selector10/1 -> Mux4/2
  Selector6/1 -> Mux3/1
  Selector7/1 -> Mux3/2
  Subsystem2/2(m_dq2) -> m_dq2/1
  [Vdc_ref] -> Subsystem2/7(Vdc_ref)
  MATLAB Function9/1 -> Reshape/1
  MATLAB Function1/1 -> Reshape1/1
  Iconv_DQN/1 -> MATLAB Function9/1
  Reshape/1 -> I->pu2/1
  Id_DQN/1 -> MATLAB Function1/1
  Reshape1/1 -> I->pu1/1
  MATLAB Function4/1 -> Reshape4/1
  Vs_DQN/1 -> MATLAB Function4/1

== system HVDC_MMC1_EMT/CTRL_DQN3 ==
  note: HRM
  note: HRM
  Vdc : Inport
  Vs_DQN : Inport  Port=2
  Iconv_DQN : Inport  Port=3
  Id_DQN : Inport  Port=4
  Demux1 : Demux  Outputs=[HrmOrd+1, HrmOrd+1, HrmOrd+1, HrmOrd+1, HrmOrd+1, HrmOrd+1]
  Demux2 : Demux  Outputs=[HrmOrd+1, HrmOrd+1, HrmOrd+1, HrmOrd+1, HrmOrd+1, HrmOrd+1]
  Demux4 : Demux  Outputs=[HrmOrd+1, HrmOrd+1, HrmOrd+1, HrmOrd+1, HrmOrd+1, HrmOrd+1]
  I->pu1 : Gain  Gain=1/Ib_ac  SaturateOnIntegerOverflow=on  OutDataTypeStr=Inherit: Same as input  ParamDataTypeStr=Inherit: Same as input
  I->pu13 : Gain  Gain=1/Vb_ac  SaturateOnIntegerOverflow=on  OutDataTypeStr=Inherit: Same as input  ParamDataTypeStr=Inherit: Same as input
  I->pu2 : Gain  Gain=1/Ib_ac  SaturateOnIntegerOverflow=on  OutDataTypeStr=Inherit: Same as input  ParamDataTypeStr=Inherit: Same as input
  Mux1 : Mux  Inputs=2
  Mux3 : Mux  Inputs=2
  Mux4 : Mux  Inputs=2
  Selector1 : Selector  InputPortWidth=HrmOrd+1  IndexOptions=Index vector (dialog)  Indices=3  OutputSizes=1
  Selector{6..7,9..10} (4 alike) : Selector  InputPortWidth=HrmOrd+1  IndexOptions=Index vector (dialog)  Indices=2  OutputSizes=1
  Selector2 : Selector  InputPortWidth=HrmOrd+1  IndexOptions=Index vector (dialog)  Indices=3  OutputSizes=1
  Subsystem1 : Subsystem  Commented=on
  Subsystem2 : Subsystem  mask{Ts=Ts_DQN, Fnom=Fnom, acdcV=acdcV, Fn_filter=Fn_filter, Zeta_filter=Zeta_filter, Kp_Preg=Kp_Preg, Ki_Preg=Ki_Preg, Limits_Preg_1=Limits_Preg(1), Limits_Preg_2=Limits_Preg(2), Kp_Qreg=Kp_Qreg, Ki_Qreg=Ki_Qreg, Limits_Qreg_1=Limits_Qreg(1), Limits_Qreg_2=Limits_Qreg(2), Kp_VDCreg=Kp_VDCreg, Ki_VDCreg=Ki_VDCreg, Limits_VDCreg_1=Limits_VDCreg(1), Limits_VDCreg_2=Limits_VDCreg(2), Kp_Ireg=Kp_Ireg, Ki_Ireg=Ki_Ireg, Limits_Ireg=Limits_Ireg, Rff=Rff, Lff=Lff, Kp_CCSC=Kp_CCSC, Ki_CCSC=Ki_CCSC}
      mask prompts: Ts "Sample time:"; Fnom "Fundamental frequency (Hz):"; Fn_filter "Natural frequency fn (Hz):"; Zeta_filter "Damping ratio Zeta"; Kp_Preg "Proportional (P):"; Ki_Preg "Integral (I):"; Limits_Preg_1 "Upper limit:"; Limits_Preg_2 "Lower limit:"; Kp_Qreg "Proportional (P):"; Ki_Qreg "Integral (I):"; Limits_Qreg_1 "Upper limit:"; Limits_Qreg_2 "Lower limit:"; Kp_VDCreg "Proportional (P):"; Ki_VDCreg "Integral (I):"; Limits_VDCreg_1 "Upper limit:"; Limits_VDCreg_2 "Lower limit:"; Kp_Ireg "Proportional (P):"; Ki_Ireg "Integral (I):"; Limits_Ireg "Output limits:"; Kp_CCSC "Proportional (P):"; Ki_CCSC "Integral (I):"
      mask DialogControl Container6 Prompt: General
      mask DialogControl Container14 Prompt: Filter
      mask DialogControl Container14_copy Prompt: Active power regulator
      mask DialogControl Container14_copy_copy Prompt: Reactive power regulator
      mask DialogControl Container14_copy_copy_copy Prompt: DC voltage regulator
      mask DialogControl Container14_copy_copy_copy_copy Prompt: Current regulator
      mask DialogControl Container14_copy_copy_copy_copy_copy Prompt: CCSC
  V->pu1 : Gain  Gain=1/Vb_ac  SaturateOnIntegerOverflow=on  OutDataTypeStr=Inherit: Same as input  ParamDataTypeStr=Inherit: Same as input
  m_dq1 : Outport
  m_dq2 : Outport  Port=2
  wires:
  Demux1/4 -> Selector10/1
  Demux4/1 -> Selector6/1
  Demux4/4 -> Selector7/1
  Demux1/1 -> Selector9/1
  V->pu1/1 -> Demux1/1
  Vs_DQN/1 -> V->pu1/1
  Id_DQN/1 -> I->pu1/1
  Vdc/1 -> I->pu13/1
  Iconv_DQN/1 -> I->pu2/1
  Subsystem2/1(m_dq1) -> m_dq1/1
  I->pu2/1 -> Demux4/1
  I->pu13/1 -> Subsystem2/1(Vdc)
  Mux4/1 -> Subsystem2/2(Vs_dq1)
  Mux3/1 -> Subsystem2/3(Iconv_dq1)
  Demux2/5 -> Selector2/1
  I->pu1/1 -> Demux2/1
  Selector1/1 -> Mux1/1
  Selector2/1 -> Mux1/2
  Mux1/1 -> Subsystem2/4(Id_dq2)
  Demux2/2 -> Selector1/1
  [PSCC_On] -> Subsystem2/8(PQreg_On1)
  [PQreg_On] -> Subsystem2/5(PQreg_On)
  [VDCreg_On] -> Subsystem2/6(VDCreg_On)
  Selector9/1 -> Mux4/1
  Selector10/1 -> Mux4/2
  Selector6/1 -> Mux3/1
  Selector7/1 -> Mux3/2
  Subsystem2/2(m_dq2) -> m_dq2/1
  [Vdc_ref] -> Subsystem2/7(Vdc_ref)

== system HVDC_MMC1_EMT/DC Circuit1 ==
  note: Cable
      | (simplified model)
  Current Measurement2 : spsCurrentMeasurementLib/Current Measurement  PhasorSimulation=off  OutputType=Complex  PSBequivalent=0
  Ground : spsGroundLib/Ground  LConnTagsString=a
  Ground2 : spsGroundLib/Ground  LConnTagsString=a
  Parallel RLC Branch{,1..3} (4 alike) : spsParallelRLCBranchLib/Parallel RLC Branch  LConnTagsString=a  RConnTagsString=__new0  BranchType=RC  Resistance=DC_cable_R_shunt  Inductance=1e-3  SetiL0=off  InitialCurrent=0  Capacitance=DC_cable_C_shunt  Setx0=off  InitialVoltage=0  Measurements=None
  Voltage Measurement2 : spsVoltageMeasurementLib/Voltage Measurement  PhasorSimulation=off  OutputType=Complex  PSBequivalent=0
  Voltage Measurement3 : spsVoltageMeasurementLib/Voltage Measurement  PhasorSimulation=off  OutputType=Complex  PSBequivalent=0
  Zcable1_1 : spsSeriesRLCBranchLib/Series RLC Branch  LConnTagsString=__new0  RConnTagsString=__new0  BranchType=RL  Resistance=R_cable  Inductance=L_cable  SetiL0=off  InitialCurrent=0  Capacitance=1e-6  Setx0=off  InitialVoltage=0  Measurements=None
  Zcable2_1 : spsSeriesRLCBranchLib/Series RLC Branch  LConnTagsString=__new0  RConnTagsString=__new0  BranchType=RL  Resistance=R_cable  Inductance=L_cable  SetiL0=off  InitialCurrent=0  Capacitance=1e-6  Setx0=off  InitialVoltage=0  Measurements=None
  CBL_plus : PMIOPort  Side=Left
  CBL_minus : PMIOPort  Port=2  Side=Left
  CBR_plus : PMIOPort  Port=3  Side=Right
  CBR_minus : PMIOPort  Port=4  Side=Right
  tag scope: Idc1=global, Vdc1=global, Vdc2=global
  wires:
  Voltage Measurement2/1 -> [Vdc1]
  Current Measurement2/1 -> [Idc1]
  Voltage Measurement3/1 -> [Vdc2]
  connections:
  CBL_minus/RConn1 -- Voltage Measurement2/LConn2 -- Zcable2_1/RConn1 -- Parallel RLC Branch1/RConn1
  Zcable1_1/RConn1 -- Voltage Measurement2/LConn1 -- Current Measurement2/LConn1 -- Parallel RLC Branch/LConn1
  Current Measurement2/RConn1 -- CBL_plus/RConn1
  Voltage Measurement3/LConn2 -- Zcable2_1/LConn1 -- CBR_minus/RConn1 -- Parallel RLC Branch3/RConn1
  Parallel RLC Branch/RConn1 -- Ground/LConn1 -- Parallel RLC Branch1/LConn1
  Parallel RLC Branch2/RConn1 -- Ground2/LConn1 -- Parallel RLC Branch3/LConn1
  Voltage Measurement3/LConn1 -- Zcable1_1/LConn1 -- CBR_plus/RConn1 -- Parallel RLC Branch2/LConn1

== system HVDC_MMC1_EMT/DC_ABC ==
  Idc1 : Inport
  Add1 : Sum  Inputs=-+
  Add5 : Sum
  Constant2 : Constant  Value=DCM
  Constant3 : Constant  Value=DCM
  DC Voltage Regulator (VDCreg)2 : Subsystem
  Delay2 : Delay  DelayLength=1
  Discrete Derivative : simulink/Discrete/Discrete Derivative  Commented=on  gainval=1  ICPrevScaledInput=0.0  OutMin=[]  OutMax=[]  OutDataType=fixdt(1, 16)  OutScaling=2^-10  DoSatur=off
  Gain3 : Gain  Gain=R_cable/2
  Gain6 : Gain  Gain=L_cable/2
  I->pu3 : Gain  Gain=1/Ib_dc  SaturateOnIntegerOverflow=on  OutDataTypeStr=Inherit: Same as input  ParamDataTypeStr=Inherit: Same as input
  I->pu5 : Gain  Gain=1/Vb_dc  SaturateOnIntegerOverflow=on  OutDataTypeStr=Inherit: Same as input  ParamDataTypeStr=Inherit: Same as input
  I->pu6 : Gain  Gain=Vnom_dc  SaturateOnIntegerOverflow=on  OutDataTypeStr=Inherit: Same as input  ParamDataTypeStr=Inherit: Same as input
  Integrator : Integrator
  Multiply1 : Product
  PDC_ref2 : Step  Time=7  Before=0.8  After=0.75  SampleTime=0
  Switch2 : Switch  Criteria=u2 > Threshold  Threshold=0.5  OutDataTypeStr=double  SaturateOnIntegerOverflow=off  InputSameDT=off
  Switch4 : Switch  Criteria=u2 > Threshold  Threshold=0.5  OutDataTypeStr=double  SaturateOnIntegerOverflow=off  InputSameDT=off
  VDC_ref1 : Step  Time=13  Before=1  After=0.95  SampleTime=0
  Vdc1 : Outport  VectorParamsAs1DForOutWhenUnconnected=off
  wires:
  Idc1/1 -> I->pu3/1, Gain3/1, Gain6/1
  [Converter2_On] -> DC Voltage Regulator (VDCreg)2/3(On)
  I->pu6/1 -> Add1/2, I->pu5/1
  Delay2/1 -> I->pu6/1
  I->pu3/1 -> Multiply1/2
  Switch2/1 -> DC Voltage Regulator (VDCreg)2/2(Meas)
  DC Voltage Regulator (VDCreg)2/1(Id_ref) -> Delay2/1
  Gain6/1 -> Integrator/1  "dVp_M"
  VDC_ref1/1 -> Switch4/1
  Gain3/1 -> Add5/2  "dVp_M"
  Multiply1/1 -> Switch2/3
  Switch4/1 -> DC Voltage Regulator (VDCreg)2/1(Ref)
  Constant2/1 -> Switch2/2
  I->pu5/1 -> Multiply1/1, Switch2/1
  Constant3/1 -> Switch4/2
  PDC_ref2/1 -> Switch4/3
  Add5/1 -> Add1/1
  Integrator/1 -> Add5/1
  Add1/1 -> Vdc1/1

== system HVDC_MMC1_EMT/DC_ABC1 ==
  Idc1 : Inport
  Add1 : Sum  Inputs=-+
  Add5 : Sum
  Constant2 : Constant  Value=DCM
  Constant3 : Constant  Value=DCM
  DC Voltage Regulator (VDCreg)2 : Subsystem
  Delay2 : Delay  DelayLength=1  SampleTime=Ts_DQN
  Discrete-Time Integrator : DiscreteIntegrator  IntegratorMethod=Accumulation: Trapezoidal  SampleTime=Ts_DQN  ICPrevOutput=DiscIntNeverNeededParam  ICPrevScaledInput=DiscIntNeverNeededParam
  Gain3 : Gain  Gain=R_cable/2
  Gain6 : Gain  Gain=L_cable/2
  I->pu3 : Gain  Gain=1/Ib_dc  SaturateOnIntegerOverflow=on  OutDataTypeStr=Inherit: Same as input  ParamDataTypeStr=Inherit: Same as input
  I->pu5 : Gain  Gain=1/Vb_dc  SaturateOnIntegerOverflow=on  OutDataTypeStr=Inherit: Same as input  ParamDataTypeStr=Inherit: Same as input
  I->pu6 : Gain  Gain=Vnom_dc  SaturateOnIntegerOverflow=on  OutDataTypeStr=Inherit: Same as input  ParamDataTypeStr=Inherit: Same as input
  Multiply1 : Product
  PDC_ref2 : Step  Time=7  Before=0.8  After=0.75  SampleTime=0
  Switch2 : Switch  Criteria=u2 > Threshold  Threshold=0.5  OutDataTypeStr=double  SaturateOnIntegerOverflow=off  InputSameDT=off
  Switch4 : Switch  Criteria=u2 > Threshold  Threshold=0.5  OutDataTypeStr=double  SaturateOnIntegerOverflow=off  InputSameDT=off
  VDC_ref1 : Step  Time=13  Before=1  After=0.95  SampleTime=0
  Vdc1 : Outport  VectorParamsAs1DForOutWhenUnconnected=off
  wires:
  Idc1/1 -> I->pu3/1, Gain3/1, Gain6/1
  [Converter2_On] -> DC Voltage Regulator (VDCreg)2/3(On)
  I->pu6/1 -> Add1/2, I->pu5/1
  Delay2/1 -> I->pu6/1
  I->pu3/1 -> Multiply1/2
  Switch2/1 -> DC Voltage Regulator (VDCreg)2/2(Meas)
  DC Voltage Regulator (VDCreg)2/1(Id_ref) -> Delay2/1
  Gain6/1 -> Discrete-Time Integrator/1  "dVp_M"
  VDC_ref1/1 -> Switch4/1
  Gain3/1 -> Add5/2  "dVp_M"
  Multiply1/1 -> Switch2/3
  Switch4/1 -> DC Voltage Regulator (VDCreg)2/1(Ref)
  Constant2/1 -> Switch2/2
  I->pu5/1 -> Multiply1/1, Switch2/1
  Constant3/1 -> Switch4/2
  PDC_ref2/1 -> Switch4/3
  Add5/1 -> Add1/1
  Discrete-Time Integrator/1 -> Add5/1
  Add1/1 -> Vdc1/1

== system HVDC_MMC1_EMT/DC_ABC2 ==
  Idc1 : Inport
  Add1 : Sum  Inputs=-+
  Add5 : Sum
  Constant2 : Constant  Value=DCM
  Constant3 : Constant  Value=DCM
  DC Voltage Regulator (VDCreg)2 : Subsystem
  Delay2 : Delay  DelayLength=1  SampleTime=Ts_DQN
  Discrete-Time Integrator : DiscreteIntegrator  IntegratorMethod=Accumulation: Trapezoidal  SampleTime=Ts_DQN  ICPrevOutput=DiscIntNeverNeededParam  ICPrevScaledInput=DiscIntNeverNeededParam
  Gain3 : Gain  Gain=R_cable/2
  Gain6 : Gain  Gain=L_cable/2
  I->pu3 : Gain  Gain=1/Ib_dc  SaturateOnIntegerOverflow=on  OutDataTypeStr=Inherit: Same as input  ParamDataTypeStr=Inherit: Same as input
  I->pu5 : Gain  Gain=1/Vb_dc  SaturateOnIntegerOverflow=on  OutDataTypeStr=Inherit: Same as input  ParamDataTypeStr=Inherit: Same as input
  I->pu6 : Gain  Gain=Vnom_dc  SaturateOnIntegerOverflow=on  OutDataTypeStr=Inherit: Same as input  ParamDataTypeStr=Inherit: Same as input
  Multiply1 : Product
  PDC_ref2 : Step  Time=7  Before=0.8  After=0.75  SampleTime=0
  Switch2 : Switch  Criteria=u2 > Threshold  Threshold=0.5  OutDataTypeStr=double  SaturateOnIntegerOverflow=off  InputSameDT=off
  Switch4 : Switch  Criteria=u2 > Threshold  Threshold=0.5  OutDataTypeStr=double  SaturateOnIntegerOverflow=off  InputSameDT=off
  VDC_ref1 : Step  Time=13  Before=1  After=0.95  SampleTime=0
  Vdc1 : Outport  VectorParamsAs1DForOutWhenUnconnected=off
  wires:
  Idc1/1 -> I->pu3/1, Gain3/1, Gain6/1
  [Converter2_On] -> DC Voltage Regulator (VDCreg)2/3(On)
  I->pu6/1 -> Add1/2, I->pu5/1
  Delay2/1 -> I->pu6/1
  I->pu3/1 -> Multiply1/2
  Switch2/1 -> DC Voltage Regulator (VDCreg)2/2(Meas)
  DC Voltage Regulator (VDCreg)2/1(Id_ref) -> Delay2/1
  Gain6/1 -> Discrete-Time Integrator/1  "dVp_M"
  VDC_ref1/1 -> Switch4/1
  Gain3/1 -> Add5/2  "dVp_M"
  Multiply1/1 -> Switch2/3
  Switch4/1 -> DC Voltage Regulator (VDCreg)2/1(Ref)
  Constant2/1 -> Switch2/2
  I->pu5/1 -> Multiply1/1, Switch2/1
  Constant3/1 -> Switch4/2
  PDC_ref2/1 -> Switch4/3
  Add5/1 -> Add1/1
  Discrete-Time Integrator/1 -> Add5/1
  Add1/1 -> Vdc1/1
